simulink model "TestConnExample"  (R2018b)
settings: Solver=FixedStepAuto  StartTime=0.0  StopTime=inf  RelTol=1e-3  EnableMultiTasking=on
libraries: px4lib x3, simulink x2, px4Sensorslib x1
settings Model: ExtModeTrigDuration=10  Creator=asheshad  LastModifiedBy=abose
settings SolverCC: PositivePriorityOrder=on
settings DataIOCC: ReturnWorkspaceOutputs=on
settings OptimizationCC: EnhancedBackFolding=on  PassReuseOutputArgsAs=Individual arguments  MaxStackSize=64  OptimizeBlockOrder=speed  DifferentSizesBufferReuse=on  OptimizationCustomize=off
settings DebuggingCC: InheritedTsInSrcMsg=none  ParameterTunabilityLossMsg=error
settings HardwareCC: ProdBitPerPointer=32  ProdBitPerSizeT=32  ProdBitPerPtrDiffT=32  ProdLargestAtomicInteger=Long  ProdLargestAtomicFloat=Double  ProdWordSize=32  ProdLongLongMode=on  ProdHWDeviceType=ARM Compatible->ARM Cortex
settings SFSimCC: MATLABDynamicMemAlloc=off
settings RTWCC: SystemTargetFile=ert.tlc  HardwareBoard=PX4 Pixhawk Series  TLCOptions="-aInlineSetEventsForThisBaseRateFcn=TLC_FALSE -aSuppressMultiTaskScheduler=TLC_FALSE  -aRateBasedStepFcn=0"  TemplateMakefile=ert_default_tmf  Toolchain=GNU Tools for PX4 Autopilots  IncludeHyperlinkInReport=on  TargetLang=C++
settings CodeAppCC: ForceParamTrailComments=on  IgnoreCustomStorageClasses=off  OperatorAnnotations=on  SimulinkDataObjDesc=on  SFDataObjDesc=on  InsertBlockDesc=on
settings ERTTargetCC: SupportVariableSizeSignals=on

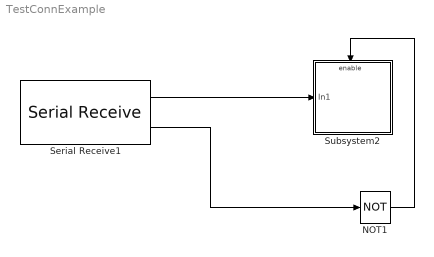
== system TestConnExample ==
  NOT1 : Logic  Operator=NOT  IconShape=distinctive  AllPortsSameDT=off  OutDataTypeStr=boolean
  Serial Receive1 : px4lib/Serial Receive  SCIModule=/dev/ttyACM0  DataType=uint8  DataLength=10  OutputStatus=on  SampleTime=0.1  BlockingMode=off  PartialData=off  Timeout=5
      settings: SourceProductName=Embedded Coder Support Package for PX4 Autopilots  SourceProductBaseCode=PX4AUTOPILOTS
  Subsystem2 : Subsystem
  wires:
  Serial Receive1/2 -> NOT1/1
  Serial Receive1/1 -> Subsystem2/1(In1)
  NOT1/1 -> Subsystem2/Enable

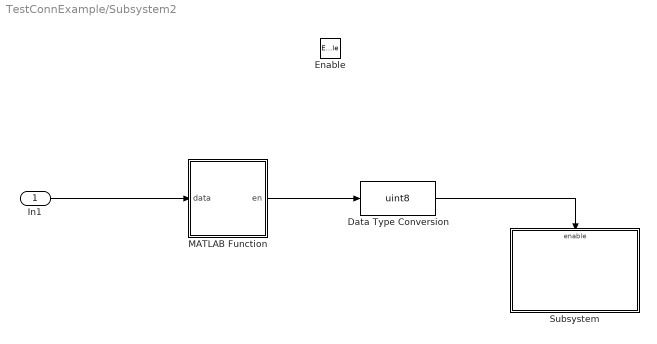
== system TestConnExample/Subsystem2 ==
  In1 : Inport
  Enable : EnablePort
  Data Type Conversion : DataTypeConversion  OutDataTypeStr=uint8
  MATLAB Function : MATLAB Function  TreatAsAtomicUnit=on
  Subsystem : Subsystem
  wires:
  In1/1 -> MATLAB Function/1(data)
  MATLAB Function/1(en) -> Data Type Conversion/1
  Data Type Conversion/1 -> Subsystem/Enable

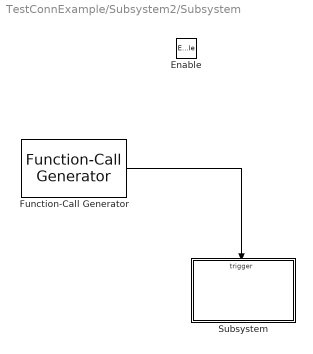
== system TestConnExample/Subsystem2/Subsystem ==
  Enable : EnablePort
  Function-Call Generator : simulink/Ports & Subsystems/Function-Call Generator  sample_time=-1  numberOfIterations=10
  Subsystem : Subsystem
  wires:
  Function-Call Generator/1 -> Subsystem/Trigger

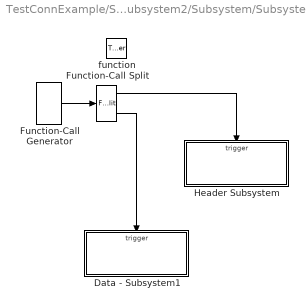
== system TestConnExample/Subsystem2/Subsystem/Subsystem ==
  function : TriggerPort  TriggerType=function-call  VariantControl=Variant
  Data - Subsystem1 : Subsystem  TreatAsAtomicUnit=on
  Function-Call Generator : simulink/Ports & Subsystems/Function-Call Generator  sample_time=-1  numberOfIterations=1
  Function-Call Split : FunctionCallSplit  IconShape=distinctive  NumOutputPorts=2  OutputPortLayout=default
  Header Subsystem : Subsystem  TreatAsAtomicUnit=on
  wires:
  Function-Call Split/2 -> Data - Subsystem1/Trigger
  Function-Call Split/1 -> Header Subsystem/Trigger
  Function-Call Generator/1 -> Function-Call Split/1

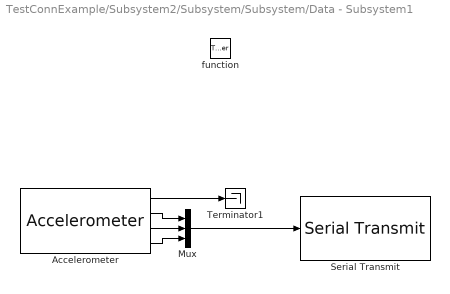
== system TestConnExample/Subsystem2/Subsystem/Subsystem/Data - Subsystem1 ==
  function : TriggerPort  TriggerType=function-call  VariantControl=Variant
  Accelerometer : px4Sensorslib/Accelerometer  uorbTimeStamp=off  BlockingMode=off  BlockTimeout=1e-3  sampleTime=-1
      settings: SourceProductName=Embedded Coder Support Package for PX4 Autopilots
  Mux : Mux  Inputs=3
  Serial Transmit : px4lib/Serial Transmit  SCIModule=/dev/ttyACM0
      settings: SourceProductName=Embedded Coder Support Package for PX4 Autopilots  SourceProductBaseCode=PX4AUTOPILOTS
  Terminator1 : Terminator
  wires:
  Mux/1 -> Serial Transmit/1
  Accelerometer/1 -> Terminator1/1
  Accelerometer/3 -> Mux/2
  Accelerometer/2 -> Mux/1
  Accelerometer/4 -> Mux/3

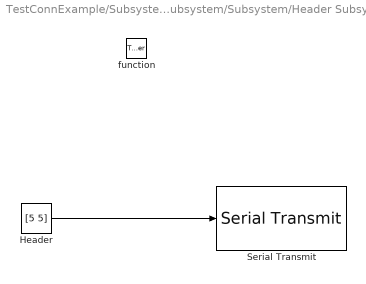
== system TestConnExample/Subsystem2/Subsystem/Subsystem/Header Subsystem ==
  function : TriggerPort  TriggerType=function-call  VariantControl=Variant
  Header : Constant  Value=[5 5]  OutDataTypeStr=uint8  SampleTime=-1
  Serial Transmit : px4lib/Serial Transmit  SCIModule=/dev/ttyACM0
      settings: SourceProductName=Embedded Coder Support Package for PX4 Autopilots  SourceProductBaseCode=PX4AUTOPILOTS
  wires:
  Header/1 -> Serial Transmit/1

== matlab function TestConnExample/Subsystem2/MATLAB Function ==
  data: data input; en output
function en  = fcn(data)
data = data';
start = [];
packet = uint8(zeros(1,3));
% data = double(data);
packetfound = false;
signaturePacket = uint8([9 9 9]);
pattern = [7 7];
% Let's assume for now that both the pattern and the array are non-empty
% VECTORS, but there's no checking for this.
% For this algorithm, I loop over the pattern elements.
len = length(pattern);
% First, find candidate locations; i.e., match the first element in the
% pattern.
start = find(data==pattern(1));
% Next remove start values that are too close to the end to possibly match
% the pattern.
endVals = start+len-1;
start(endVals>length(data)) = [];
% Next, loop over elements of pattern, usually much shorter than length of
% array, to check which possible locations are valid still.
for pattval = 2:len
    % check viable locations in array
    locs = pattern(pattval) == data(start+pattval-1);
    % delete false ones from indices
    start(~locs) = [];
end

expectedPacketSize = 5;

if ~isempty(start)
    for i = 1:length(start)
        if isequal(start(i+1)-start(i),expectedPacketSize)
            packet = data(start(i)+2:start(i+1)-1);
            if ~isequal(length(packet),(expectedPacketSize-length(pattern)))
                error('ERROR:Wrong packet size');
            end
            packetfound = true;
            break;
        else
            continue
        end
    end
else
    packetfound = false;
end

if packetfound && isequal(packet,signaturePacket)
    en = 1;
else
    en = 0;
end

end
